simulink subsystem "s1EMSSC"  (R2024a)
settings: Solver=VariableStepAuto  StartTime=0.0  StopTime=10.0  RelTol=1e-3
undefined symbols (not defined in the file): HVDCNeg, HVDCPos
libraries: fl_lib x7, nesl_utility_internal x4, nesl_utility x1
settings Model: ModifiedByFormat=The MathWorks, Inc.  Creator=The MathWorks, Inc.  LastModifiedBy=The MathWorks, Inc.
settings RTWCC: GPUComputeCapability=3.5

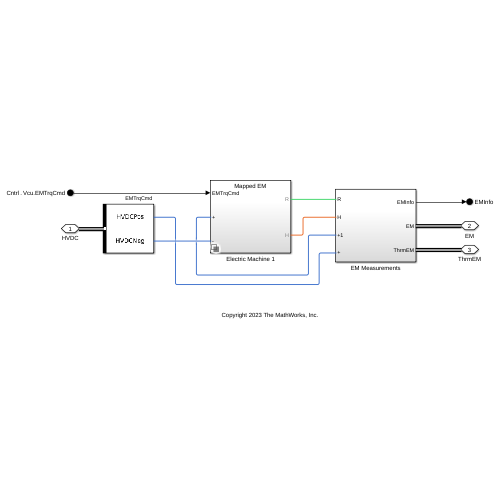
[thumbnail: Simulink's stored preview of the top-level diagram]
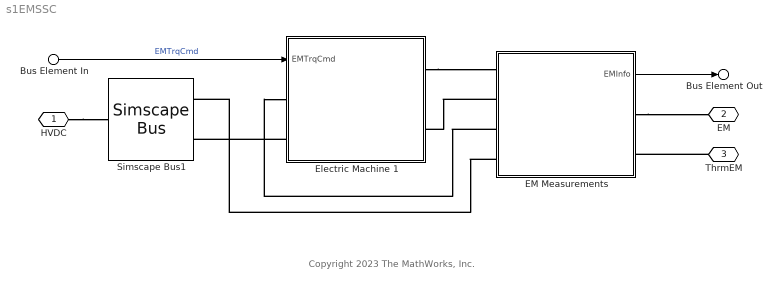
== system s1EMSSC ==
  note: Copyright 2023 The MathWorks, Inc.
  Bus Element In : Inport  PortName=Cntrl  Element=Vcu.EMTrqCmd
  EM Measurements : Subsystem
  Electric Machine 1 : Subsystem  Variant=on  VariantControlMode=label  LabelModeActiveChoice=Mapped EM
  Simscape Bus1 : SimscapeBus  HierarchyStrings=HVDCPos;HVDCNeg
  HVDC : PMIOPort  Side=Left
  EM : PMIOPort  Port=2  Side=Right
  ThrmEM : PMIOPort  Port=3  Side=Right
  Bus Element Out : Outport  PortName=EMInfo
  wires:
  Bus Element In/1 -> Electric Machine 1/1(EMTrqCmd)  "EMTrqCmd"
  EM Measurements/1(EMInfo) -> Bus Element Out/1
  connections:
  HVDC/RConn1 -- Simscape Bus1/RConn1
  EM Measurements/LConn4 -- Simscape Bus1/LConn1
  Electric Machine 1/LConn2 -- Simscape Bus1/LConn2
  Electric Machine 1/RConn1 -- EM Measurements/LConn1
  EM Measurements/RConn1 -- EM/RConn1
  EM Measurements/LConn2 -- Electric Machine 1/RConn2
  ThrmEM/RConn1 -- EM Measurements/RConn2
  EM Measurements/LConn3 -- Electric Machine 1/LConn1

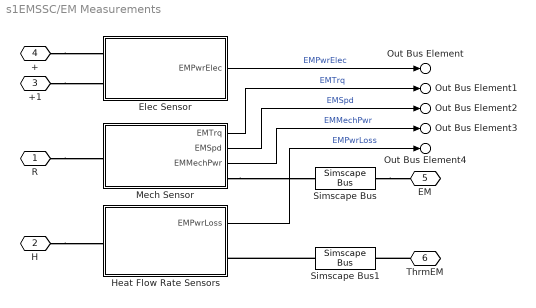
== system s1EMSSC/EM Measurements ==
  Elec Sensor : Subsystem
  Heat Flow Rate Sensors : Subsystem
  Mech Sensor : Subsystem
  Simscape Bus : SimscapeBus  HierarchyStrings=EM1
  Simscape Bus1 : SimscapeBus  HierarchyStrings=ThrmEM1
  R : PMIOPort  Side=Left
  H : PMIOPort  Port=2  Side=Left
  +1 : PMIOPort  Port=3  Side=Left
  + : PMIOPort  Port=4  Side=Left
  EM : PMIOPort  Port=5  Side=Right
  ThrmEM : PMIOPort  Port=6  Side=Right
  Out Bus Element : Outport  PortName=EMInfo  Element=EMPwrElec
  Out Bus Element1 : Outport  PortName=EMInfo  Element=EMTrq
  Out Bus Element2 : Outport  PortName=EMInfo  Element=EMSpd
  Out Bus Element3 : Outport  PortName=EMInfo  Element=EMMechPwr
  Out Bus Element4 : Outport  PortName=EMInfo  Element=EMPwrLoss
  wires:
  Mech Sensor/3(EMMechPwr) -> Out Bus Element3/1  "EMMechPwr"
  Mech Sensor/2(EMSpd) -> Out Bus Element2/1  "EMSpd"
  Mech Sensor/1(EMTrq) -> Out Bus Element1/1  "EMTrq"
  Elec Sensor/1(EMPwrElec) -> Out Bus Element/1  "EMPwrElec"
  Heat Flow Rate Sensors/1(EMPwrLoss) -> Out Bus Element4/1  "EMPwrLoss"
  connections:
  Simscape Bus1/LConn1 -- Heat Flow Rate Sensors/RConn1
  H/RConn1 -- Heat Flow Rate Sensors/LConn1
  +1/RConn1 -- Elec Sensor/LConn2
  +/RConn1 -- Elec Sensor/LConn1
  R/RConn1 -- Mech Sensor/LConn1
  Mech Sensor/RConn1 -- Simscape Bus/LConn1
  ThrmEM/RConn1 -- Simscape Bus1/RConn1
  Simscape Bus/RConn1 -- EM/RConn1

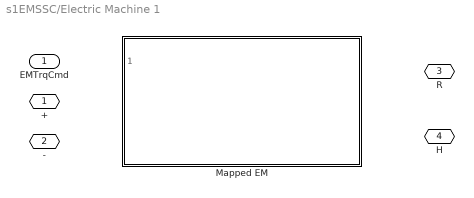
== system s1EMSSC/Electric Machine 1 ==
  EMTrqCmd : Inport
  Mapped EM : Subsystem  VariantControl=Mapped EM  ReferencedSubsystem=ElectricMachine1SSC
  + : PMIOPort  Side=Left
  - : PMIOPort  Port=2  Side=Left
  R : PMIOPort  Port=3  Side=Right
  H : PMIOPort  Port=4  Side=Right

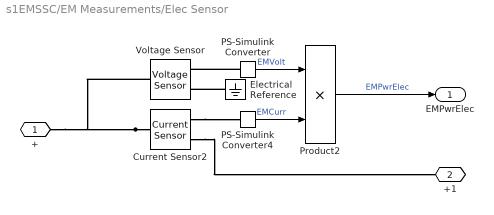
== system s1EMSSC/EM Measurements/Elec Sensor ==
  Current Sensor2 : fl_lib/Electrical/Electrical Sensors/Current Sensor
  Electrical Reference : fl_lib/Electrical/Electrical Elements/Electrical Reference
  PS-Simulink Converter : nesl_utility_internal/PS-Simulink Converter  PhysicalDomain=network_engine_domain  SubClassName=ps_output  LeftPortType=input  RightPortType=output  PseudoPeriodic=off  Frequencies=[]  VectorFormat=1-D array  Unit=inherit  AffineConversion=off
  PS-Simulink Converter4 : nesl_utility_internal/PS-Simulink Converter  PhysicalDomain=network_engine_domain  SubClassName=ps_output  LeftPortType=input  RightPortType=output  PseudoPeriodic=off  Frequencies=[]  VectorFormat=1-D array  Unit=1  AffineConversion=off
  Product2 : Product
  Voltage Sensor : fl_lib/Electrical/Electrical Sensors/Voltage Sensor
  + : PMIOPort  Side=Left
  +1 : PMIOPort  Port=2  Side=Left
  EMPwrElec : Outport
  wires:
  PS-Simulink Converter/1 -> Product2/1  "EMVolt"
  Product2/1 -> EMPwrElec/1  "EMPwrElec"
  PS-Simulink Converter4/1 -> Product2/2  "EMCurr"
  connections:
  PS-Simulink Converter/LConn1 -- Voltage Sensor/RConn1
  Electrical Reference/LConn1 -- Voltage Sensor/RConn2
  Current Sensor2/LConn1 -- Voltage Sensor/LConn1 -- +/RConn1
  Current Sensor2/RConn2 -- +1/RConn1
  Current Sensor2/RConn1 -- PS-Simulink Converter4/LConn1

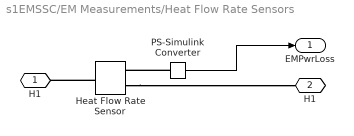
== system s1EMSSC/EM Measurements/Heat Flow Rate Sensors ==
  Heat Flow Rate Sensor : fl_lib/Thermal/Thermal Sensors/Heat Flow Rate Sensor
  PS-Simulink Converter : nesl_utility/PS-Simulink Converter  PhysicalDomain=network_engine_domain  SubClassName=ps_output  LeftPortType=input  RightPortType=output  PseudoPeriodic=off  Frequencies=[]  VectorFormat=inherit  Unit=inherit  AffineConversion=off
  H1 : PMIOPort  Side=Left
  "H1 " : PMIOPort  Port=2  Side=Right
  EMPwrLoss : Outport
  wires:
  PS-Simulink Converter/1 -> EMPwrLoss/1
  connections:
  Heat Flow Rate Sensor/LConn1 -- H1/RConn1
  Heat Flow Rate Sensor/RConn2 -- "H1 "/RConn1
  PS-Simulink Converter/LConn1 -- Heat Flow Rate Sensor/RConn1

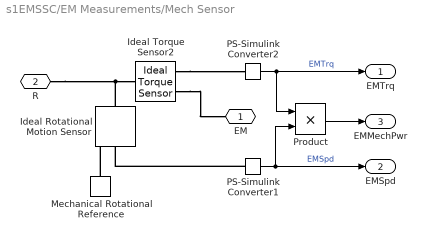
== system s1EMSSC/EM Measurements/Mech Sensor ==
  Ideal Rotational Motion Sensor : fl_lib/Mechanical/Mechanical Sensors/Ideal Rotational Motion Sensor  reference=foundation.enum.MeasurementReference.difference  acceleration_port=false  velocity_port=true  position_port=true  wrap_angle=false  offset=0 rad
  Ideal Torque Sensor2 : fl_lib/Mechanical/Mechanical Sensors/Ideal Torque Sensor
  Mechanical Rotational Reference : fl_lib/Mechanical/Rotational Elements/Mechanical Rotational Reference
  PS-Simulink Converter1 : nesl_utility_internal/PS-Simulink Converter  PhysicalDomain=network_engine_domain  SubClassName=ps_output  LeftPortType=input  RightPortType=output  PseudoPeriodic=off  Frequencies=[]  VectorFormat=1-D array  Unit=rad/s  AffineConversion=off
  PS-Simulink Converter2 : nesl_utility_internal/PS-Simulink Converter  PhysicalDomain=network_engine_domain  SubClassName=ps_output  LeftPortType=input  RightPortType=output  PseudoPeriodic=off  Frequencies=[]  VectorFormat=1-D array  Unit=1  AffineConversion=off
  Product : Product
  EM : PMIOPort  Side=Right
  R : PMIOPort  Port=2  Side=Left
  EMTrq : Outport
  EMSpd : Outport  Port=2
  EMMechPwr : Outport  Port=3
  wires:
  Product/1 -> EMMechPwr/1
  PS-Simulink Converter1/1 -> EMSpd/1, Product/2  "EMSpd"
  PS-Simulink Converter2/1 -> EMTrq/1, Product/1  "EMTrq"
  connections:
  PS-Simulink Converter1/LConn1 -- Ideal Rotational Motion Sensor/RConn2
  Mechanical Rotational Reference/LConn1 -- Ideal Rotational Motion Sensor/RConn1
  Ideal Torque Sensor2/RConn1 -- EM/RConn1
  Ideal Rotational Motion Sensor/LConn1 -- R/RConn1 -- Ideal Torque Sensor2/LConn1
  Ideal Torque Sensor2/RConn2 -- PS-Simulink Converter2/LConn1
